simulink model "SystemModel"  (Simulink 8.6)
settings: Solver=ode45  StartTime=0.0  StopTime=25  RelTol=1e-3
values from neighbouring files (symbols this model uses):
  Alt = [ 00  03  03  18  18  05  00  00 ... (first row only)    [constants.m]
  ControlDriverGain = 4.8    [setup.m]
  CurrentDriverBias = Vss/2    [setup.m]
  mBackEMF = 1/Kbmm    [setup.m]
  mElecDynDen = [Lmm Rmm]    [setup.m]
  mElecDynNum = [1]    [setup.m]
  mHeliDynDen = [M B1 0]    [setup.m]
  mHeliDynNum = [0 0 1]    [setup.m]
  mMechDynDen = [Jmm+Jmr Bmm+Bmr]    [setup.m]
  mMechDynNum = [RPMPerw / Kgm2Pergcm2]    [setup.m]
  mPID = [0.0446, 0.0497, 0.0388]    [setup.m]
  mSat = Vss/2    [setup.m]
  mTConst = Ktmm    [setup.m]
  potentiometerBias = Vss/2    [setup.m]
  potentiometerGain = Vss/(2*angleRange)    [setup.m]
  tHeliDynDen = [Jh B2h 0] * Kgm2Pergcm2    [setup.m]
  tHeliDynNum = [0 0 1]    [setup.m]
  torqueFromAltMotorMass = (mainBracketMass + Mmm) * G * mainArmLength    [setup.m]
  torqueFromYawMotorMass = (tailBracketMass + Mtm) * G * yawArmLength    [setup.m]
  tSat = Vss/2    [setup.m]
  tTorque = TPtr*1e-6 * G * Lh*1e-2 * Ntr    [setup.m]
  Yaw = [ 00  00  60  60 180 180 ... (first row only)    [constants.m]
undefined symbols (not defined in the file or in its folder): mLift
libraries: simulink x4, vrlib x1, simulink_extras x1
settings Model: Creator=Leos  LastModifiedBy=Wyatt
settings DataIOCC: LimitDataPoints=off
settings DebuggingCC: FcnCallInpInsideContextMsg=UseLocalSettings
settings ConfigComp: CovSFcnEnable=off

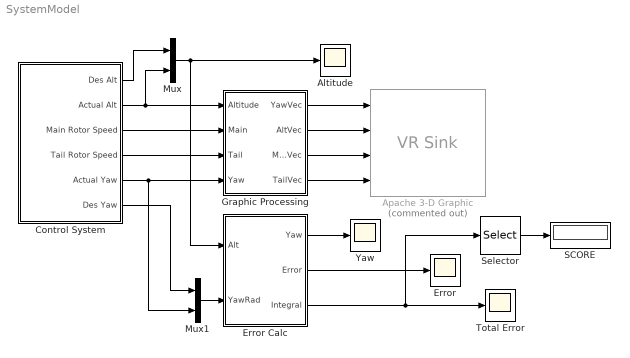
== system SystemModel ==
  Altitude : Scope
  Apache 3-D Graphic : vrlib/VR Sink  Commented=on  InstantiateOnLoad=on  SampleTime=-1  ViewEnable=on  RemoteChange=off  RemoteView=off  FieldsWritten=Helicopter.rotation.4.1.double#Helicopter.translation.3.1.double#Main.rotation.4.1.double#Tail.rotation.4.1.double  WorldFileName=Apache.WRL  AutoView=on  VideoDimensions=[]  AllowVariableSize=off  FigureProperties="{'Position', 'Name', 'Viewpoint', 'CameraBound', 'CameraDirection', 'CameraPosition', 'CameraUpVector', 'ZoomFactor', 'Antialiasing', 'Headlight', 'Lighting', 'NavPanel', 'Sound', 'StatusBar', 'Stereo3D', 'Stereo3DCameraOffset', 'Stereo3DHIT', 'ToolBar', 'Textures', 'Transparency', 'Triad', 'Wireframe', 'NavZones', 'NavMode', 'NavSpeed', 'CaptureFileFormat', 'CaptureFileName', 'Record2DCompressMethod', 'Record2DCompressQuality', 'Record2D', 'Record2DFileName', 'Record2DFPS'; [2.7530000000000000e+03  -5.1800000000000000e+02   5.7600000000000000e+02   3.8000000000000000e+02], '', '_untitled_1', 'on', [0.0000000000000000e+00   0.0000000000000000e+00  -1.0000000000000000e+00], [0.0000000000000000e+00   0.0000000000000000e+00   0.0000000000000000e+00], [0.0000000000000000e+00   1.0000000000000000e+00   0.0000000000000000e+00], [1.0000000000000000e+00], 'on', 'on', 'on', 'halfbar', 'on', 'on', 'off', [1.0000000149011612e-01], [0.0000000000000000e+00], 'on', 'on', 'on', 'none', 'off', 'off', 'walk', 'normal', 'tif', '%f_anim_%n.tif', 'auto', [7.5000000000000000e+01], 'off', '%f_anim_%n.avi', 'auto'}"
  Control System : Subsystem
  Error : Scope
  Error Calc : Subsystem
  Graphic Processing : Subsystem
  Mux : Mux  Inputs=2
  Mux1 : Mux  Inputs=2
  SCORE : Display
  Selector : Selector  InputPortWidth=3  IndexOptions=Index vector (dialog)  Indices=[3]  OutputSizes=1
  Total Error : Scope
  Yaw : Scope
  wires:
  Mux/1 -> Error Calc/1(Alt), Altitude/1
  Control System/1(Des Alt) -> Mux/1
  Control System/2(Actual Alt) -> Mux/2, Graphic Processing/1(Altitude)
  Control System/5(Actual Yaw) -> Mux1/2, Graphic Processing/4(Yaw)
  Graphic Processing/1(YawVec) -> Apache 3-D Graphic/1
  Graphic Processing/2(AltVec) -> Apache 3-D Graphic/2
  Graphic Processing/3(MainVec) -> Apache 3-D Graphic/3
  Graphic Processing/4(TailVec) -> Apache 3-D Graphic/4
  Control System/4(Tail Rotor Speed) -> Graphic Processing/3(Tail)
  Control System/3(Main Rotor Speed) -> Graphic Processing/2(Main)
  Control System/6(Des Yaw) -> Mux1/1
  Mux1/1 -> Error Calc/2(YawRad)
  Error Calc/1(Yaw) -> Yaw/1
  Error Calc/2(Error) -> Error/1
  Error Calc/3(Integral) -> Selector/1, Total Error/1
  Selector/1 -> SCORE/1

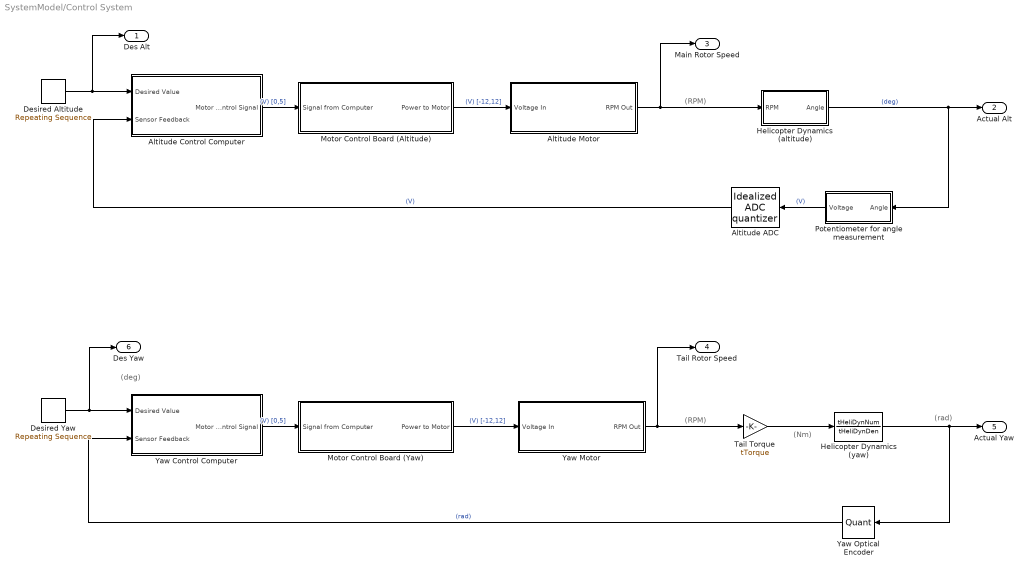
== system SystemModel/Control System ==
  note: (RPM)
  note: (deg)
  note: (RPM)
  note: (Nm)
  note: (rad)
  Altitude ADC : simulink_extras/Additional Discrete/Idealized ADC quantizer  NumberOfConverterBits=ADC_bitwidth  Vmin=ground  Vmax=Vss  OutputDataType=int16  OutputNegativeValues=off
  Altitude Control Computer : Subsystem
  Altitude Motor : Subsystem
  Desired Altitude : simulink/Sources/Repeating Sequence  rep_seq_t=Alt(2,:)  rep_seq_y=Alt(1,:)
  Desired Yaw : simulink/Sources/Repeating Sequence  rep_seq_t=Yaw(2,:)  rep_seq_y=Yaw(1,:)
  Helicopter Dynamics (yaw) : TransferFcn  Numerator=tHeliDynNum  Denominator=tHeliDynDen
  Helicopter Dynamics (altitude) : Subsystem
  Motor Control Board (Altitude) : Subsystem
  Motor Control Board (Yaw) : Subsystem
  Potentiometer for angle measurement : Subsystem
  Tail Torque : Gain  Gain=tTorque
  Yaw Control Computer : Subsystem
  Yaw Motor : Subsystem
  Yaw Optical Encoder : Quantizer  QuantizationInterval=YawEncoderQuantization
  Des Alt : Outport
  Actual Alt : Outport  Port=2
  Main Rotor Speed : Outport  Port=3
  Tail Rotor Speed : Outport  Port=4
  Actual Yaw : Outport  Port=5
  Des Yaw : Outport  Port=6
  wires:
  Desired Altitude/1 -> Altitude Control Computer/1(Desired Value), Des Alt/1
  Tail Torque/1 -> Helicopter Dynamics (yaw)/1
  Helicopter Dynamics (yaw)/1 -> Yaw Optical Encoder/1, Actual Yaw/1
  Desired Yaw/1 -> Yaw Control Computer/1(Desired Value), Des Yaw/1
  Altitude Motor/1(RPM Out) -> Helicopter Dynamics (altitude)/1(RPM), Main Rotor Speed/1
  Yaw Optical Encoder/1 -> Yaw Control Computer/2(Sensor Feedback)  "(rad)"
  Yaw Control Computer/1(Motor Driver Control Signal) -> Motor Control Board (Yaw)/1(Signal from Computer)  "(V) [0,5]"
  Altitude Control Computer/1(Motor Driver Control Signal) -> Motor Control Board (Altitude)/1(Signal from Computer)  "(V) [0,5]"
  Motor Control Board (Altitude)/1(Power to Motor) -> Altitude Motor/1(Voltage In)  "(V) [-12,12]"
  Motor Control Board (Yaw)/1(Power to Motor) -> Yaw Motor/1(Voltage In)  "(V) [-12,12]"
  Yaw Motor/1(RPM Out) -> Tail Torque/1, Tail Rotor Speed/1
  Altitude ADC/1 -> Altitude Control Computer/2(Sensor Feedback)  "(V)"
  Potentiometer for angle measurement/1(Voltage) -> Altitude ADC/1  "(V)"
  Helicopter Dynamics (altitude)/1(Angle) -> Actual Alt/1, Potentiometer for angle measurement/1(Angle)  "(deg)"

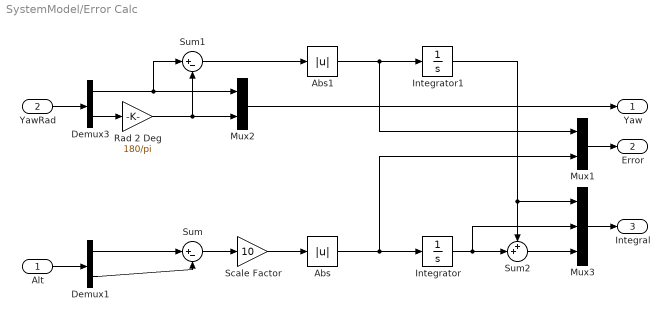
== system SystemModel/Error Calc ==
  Alt : Inport
  YawRad : Inport  Port=2
  Abs : Abs
  Abs1 : Abs
  Demux1 : Demux  Outputs=2
  Demux3 : Demux  Outputs=2
  Integrator : Integrator
  Integrator1 : Integrator
  Mux1 : Mux  Inputs=2
  Mux2 : Mux  Inputs=2
  Mux3 : Mux  Inputs=3
  Rad 2 Deg : Gain  Gain=180/pi
  Scale Factor : Gain  Gain=10
  Sum : Sum  Inputs=|+-
  Sum1 : Sum  Inputs=|+-
  Sum2 : Sum  Inputs=++|
  Yaw : Outport
  Error : Outport  Port=2
  Integral : Outport  Port=3
  wires:
  YawRad/1 -> Demux3/1
  Alt/1 -> Demux1/1
  Mux2/1 -> Yaw/1
  Rad 2 Deg/1 -> Sum1/2, Mux2/2
  Demux3/2 -> Rad 2 Deg/1
  Demux3/1 -> Sum1/1, Mux2/1
  Demux1/1 -> Sum/1
  Demux1/2 -> Sum/2
  Sum/1 -> Scale Factor/1
  Mux1/1 -> Error/1
  Sum1/1 -> Abs1/1
  Abs1/1 -> Mux1/1, Integrator1/1
  Scale Factor/1 -> Abs/1
  Abs/1 -> Mux1/2, Integrator/1
  Mux3/1 -> Integral/1
  Integrator/1 -> Mux3/2, Sum2/2
  Integrator1/1 -> Mux3/1, Sum2/1
  Sum2/1 -> Mux3/3

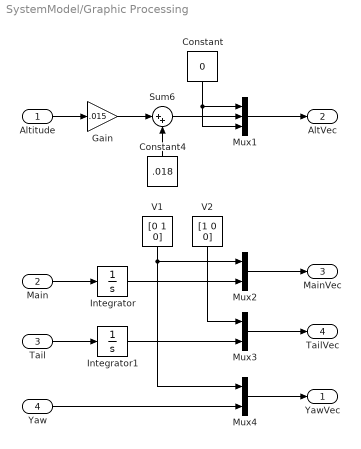
== system SystemModel/Graphic Processing ==
  Altitude : Inport
  Main : Inport  Port=2
  Tail : Inport  Port=3
  Yaw : Inport  Port=4
  Constant : Constant  Value=0
  Constant4 : Constant  Value=.018
  Gain : Gain  Gain=.015
  Integrator : Integrator
  Integrator1 : Integrator
  Mux1 : Mux  Inputs=3
  Mux2 : Mux  Inputs=2
  Mux3 : Mux  Inputs=2
  Mux4 : Mux  Inputs=2
  Sum6 : Sum  Inputs=|++
  V1 : Constant  Value=[0 1 0]
  V2 : Constant  Value=[1 0 0]
  YawVec : Outport
  AltVec : Outport  Port=2
  MainVec : Outport  Port=3
  TailVec : Outport  Port=4
  wires:
  V2/1 -> Mux3/1
  Yaw/1 -> Mux4/2
  Altitude/1 -> Gain/1
  Constant4/1 -> Sum6/2
  Sum6/1 -> Mux1/2
  Gain/1 -> Sum6/1
  Mux4/1 -> YawVec/1
  Mux3/1 -> TailVec/1
  Tail/1 -> Integrator1/1
  Mux2/1 -> MainVec/1
  Mux1/1 -> AltVec/1
  V1/1 -> Mux4/1, Mux2/1
  Main/1 -> Integrator/1
  Constant/1 -> Mux1/3, Mux1/1
  Integrator/1 -> Mux2/2
  Integrator1/1 -> Mux3/2

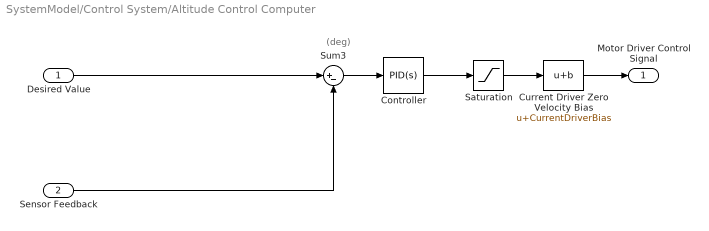
== system SystemModel/Control System/Altitude Control Computer ==
  note: (deg)
  Desired Value : Inport
  Sensor Feedback : Inport  Port=2
  Controller : simulink/Continuous/PID Controller  Controller=PID  TimeDomain=Continuous-time  SampleTime=-1  IntegratorMethod=Forward Euler  FilterMethod=Forward Euler  Form=Parallel  UseFilter=on  ControllerParametersSource=internal  P=mPID(1)  I=mPID(2)  D=mPID(3)  N=100  InitialConditionSource=internal  InitialConditionForIntegrator=0  InitialConditionForFilter=0  ExternalReset=none  LimitOutput=off  UpperSaturationLimit=inf  LowerSaturationLimit=-inf  LinearizeAsGain=on  AntiWindupMode=none  Kb=1  TrackingMode=off  Kt=1  PParamMin=[]  PParamMax=[]  IParamMin=[]  IParamMax=[]  DParamMin=[]  DParamMax=[]  NParamMin=[]  NParamMax=[]  KbParamMin=[]  KbParamMax=[]  KtParamMin=[]  KtParamMax=[]  POutMin=[]  POutMax=[]  IOutMin=[]  IOutMax=[]  DOutMin=[]  DOutMax=[]  NOutMin=[]  NOutMax=[]  KbOutMin=[]  KbOutMax=[]  KtOutMin=[]  KtOutMax=[]  IntegratorOutMin=[]  IntegratorOutMax=[]  FilterOutMin=[]  FilterOutMax=[]  SumOutMin=[]  SumOutMax=[]  SumI1OutMin=[]  SumI1OutMax=[]  SumI2OutMin=[]  SumI2OutMax=[]  SumI3OutMin=[]  SumI3OutMax=[]  SumDOutMin=[]  SumDOutMax=[]  SaturationOutMin=[]  SaturationOutMax=[]  IntegratorContinuousStateAttributes=''  IntegratorStateMustResolveToSignalObject=off  IntegratorRTWStateStorageClass=Auto  FilterContinuousStateAttributes=''  FilterStateMustResolveToSignalObject=off  FilterRTWStateStorageClass=Auto  DifferentiatorICPrevScaledInput=0  DifferentiatorOutMin=[]  DifferentiatorOutMax=[]
  Current Driver Zero Velocity Bias : Bias  Bias=CurrentDriverBias
  Saturation : Saturate  UpperLimit=mSat  LowerLimit=-mSat
  Sum3 : Sum  Inputs=|+-
  Motor Driver Control Signal : Outport
  wires:
  Desired Value/1 -> Sum3/1
  Sensor Feedback/1 -> Sum3/2
  Sum3/1 -> Controller/1
  Saturation/1 -> Current Driver Zero Velocity Bias/1
  Controller/1 -> Saturation/1
  Current Driver Zero Velocity Bias/1 -> Motor Driver Control Signal/1

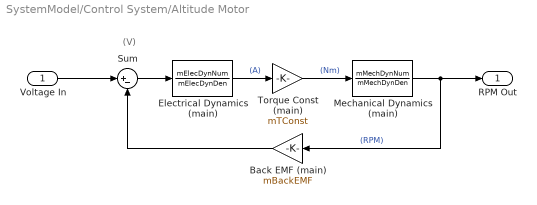
== system SystemModel/Control System/Altitude Motor ==
  note: (V)
  Voltage In : Inport
  Back EMF (main) : Gain  Gain=mBackEMF
  Electrical Dynamics (main) : TransferFcn  Numerator=mElecDynNum  Denominator=mElecDynDen
  Mechanical Dynamics (main) : TransferFcn  Numerator=mMechDynNum  Denominator=mMechDynDen
  Sum : Sum  Inputs=|+-
  Torque Const (main) : Gain  Gain=mTConst
  RPM Out : Outport
  wires:
  Voltage In/1 -> Sum/1
  Torque Const (main)/1 -> Mechanical Dynamics (main)/1  "(Nm)"
  Back EMF (main)/1 -> Sum/2
  Mechanical Dynamics (main)/1 -> RPM Out/1, Back EMF (main)/1  "(RPM)"
  Electrical Dynamics (main)/1 -> Torque Const (main)/1  "(A)"
  Sum/1 -> Electrical Dynamics (main)/1

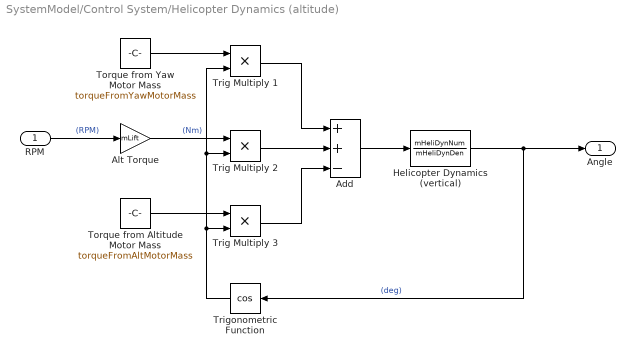
== system SystemModel/Control System/Helicopter Dynamics (altitude) ==
  RPM : Inport
  Add : Sum  Inputs=++-
  Alt Torque : Gain  Gain=mLift
  Helicopter Dynamics (vertical) : TransferFcn  Numerator=mHeliDynNum  Denominator=mHeliDynDen
  Torque from Altitude Motor Mass : Constant  Value=torqueFromAltMotorMass
  "Torque from Yaw Motor Mass " : Constant  Value=torqueFromYawMotorMass
  Trig Multiply 1 : Product
  Trig Multiply 2 : Product
  Trig Multiply 3 : Product
  Trigonometric Function : Trigonometry  Operator=cos
  Angle : Outport
  wires:
  RPM/1 -> Alt Torque/1  "(RPM)"
  Helicopter Dynamics (vertical)/1 -> Angle/1, Trigonometric Function/1  "(deg)"
  Alt Torque/1 -> Trig Multiply 2/1  "(Nm)"
  Trigonometric Function/1 -> Trig Multiply 3/2, Trig Multiply 2/2, Trig Multiply 1/2
  "Torque from Yaw Motor Mass "/1 -> Trig Multiply 1/1
  Add/1 -> Helicopter Dynamics (vertical)/1
  Trig Multiply 2/1 -> Add/2
  Trig Multiply 1/1 -> Add/1
  Torque from Altitude Motor Mass/1 -> Trig Multiply 3/1
  Trig Multiply 3/1 -> Add/3

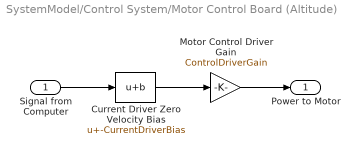
== system SystemModel/Control System/Motor Control Board (Altitude) ==
  Signal from Computer : Inport
  Current Driver Zero Velocity Bias : Bias  Bias=-CurrentDriverBias
  Motor Control Driver Gain : Gain  Gain=ControlDriverGain
  Power to Motor : Outport
  wires:
  Motor Control Driver Gain/1 -> Power to Motor/1
  Signal from Computer/1 -> Current Driver Zero Velocity Bias/1
  Current Driver Zero Velocity Bias/1 -> Motor Control Driver Gain/1

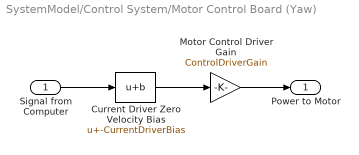
== system SystemModel/Control System/Motor Control Board (Yaw) ==
  Signal from Computer : Inport
  Current Driver Zero Velocity Bias : Bias  Bias=-CurrentDriverBias
  Motor Control Driver Gain : Gain  Gain=ControlDriverGain
  Power to Motor : Outport
  wires:
  Motor Control Driver Gain/1 -> Power to Motor/1
  Signal from Computer/1 -> Current Driver Zero Velocity Bias/1
  Current Driver Zero Velocity Bias/1 -> Motor Control Driver Gain/1

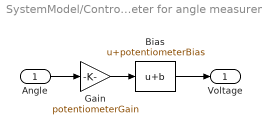
== system SystemModel/Control System/Potentiometer for angle measurement ==
  Angle : Inport
  Bias : Bias  Bias=potentiometerBias
  Gain : Gain  Gain=potentiometerGain
  Voltage : Outport
  wires:
  Bias/1 -> Voltage/1
  Angle/1 -> Gain/1
  Gain/1 -> Bias/1

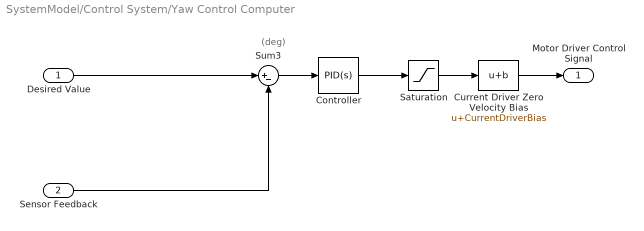
== system SystemModel/Control System/Yaw Control Computer ==
  note: (deg)
  Desired Value : Inport
  Sensor Feedback : Inport  Port=2
  Controller : simulink/Continuous/PID Controller  Controller=PID  TimeDomain=Continuous-time  SampleTime=-1  IntegratorMethod=Forward Euler  FilterMethod=Forward Euler  Form=Parallel  UseFilter=on  ControllerParametersSource=internal  P=mPID(1)  I=mPID(2)  D=mPID(3)  N=100  InitialConditionSource=internal  InitialConditionForIntegrator=0  InitialConditionForFilter=0  ExternalReset=none  LimitOutput=off  UpperSaturationLimit=inf  LowerSaturationLimit=-inf  LinearizeAsGain=on  AntiWindupMode=none  Kb=1  TrackingMode=off  Kt=1  PParamMin=[]  PParamMax=[]  IParamMin=[]  IParamMax=[]  DParamMin=[]  DParamMax=[]  NParamMin=[]  NParamMax=[]  KbParamMin=[]  KbParamMax=[]  KtParamMin=[]  KtParamMax=[]  POutMin=[]  POutMax=[]  IOutMin=[]  IOutMax=[]  DOutMin=[]  DOutMax=[]  NOutMin=[]  NOutMax=[]  KbOutMin=[]  KbOutMax=[]  KtOutMin=[]  KtOutMax=[]  IntegratorOutMin=[]  IntegratorOutMax=[]  FilterOutMin=[]  FilterOutMax=[]  SumOutMin=[]  SumOutMax=[]  SumI1OutMin=[]  SumI1OutMax=[]  SumI2OutMin=[]  SumI2OutMax=[]  SumI3OutMin=[]  SumI3OutMax=[]  SumDOutMin=[]  SumDOutMax=[]  SaturationOutMin=[]  SaturationOutMax=[]  IntegratorContinuousStateAttributes=''  IntegratorStateMustResolveToSignalObject=off  IntegratorRTWStateStorageClass=Auto  FilterContinuousStateAttributes=''  FilterStateMustResolveToSignalObject=off  FilterRTWStateStorageClass=Auto  DifferentiatorICPrevScaledInput=0  DifferentiatorOutMin=[]  DifferentiatorOutMax=[]
  Current Driver Zero Velocity Bias : Bias  Bias=CurrentDriverBias
  Saturation : Saturate  UpperLimit=tSat  LowerLimit=-tSat
  Sum3 : Sum  Inputs=|+-
  Motor Driver Control Signal : Outport
  wires:
  Desired Value/1 -> Sum3/1
  Sensor Feedback/1 -> Sum3/2
  Sum3/1 -> Controller/1
  Saturation/1 -> Current Driver Zero Velocity Bias/1
  Controller/1 -> Saturation/1
  Current Driver Zero Velocity Bias/1 -> Motor Driver Control Signal/1

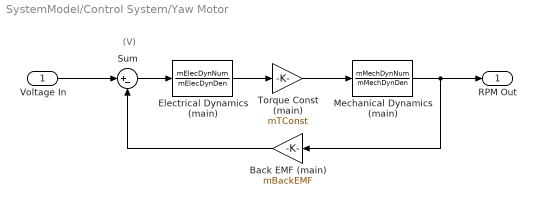
== system SystemModel/Control System/Yaw Motor ==
  note: (V)
  Voltage In : Inport
  Back EMF (main) : Gain  Gain=mBackEMF
  Electrical Dynamics (main) : TransferFcn  Numerator=mElecDynNum  Denominator=mElecDynDen
  Mechanical Dynamics (main) : TransferFcn  Numerator=mMechDynNum  Denominator=mMechDynDen
  Sum : Sum  Inputs=|+-
  Torque Const (main) : Gain  Gain=mTConst
  RPM Out : Outport
  wires:
  Voltage In/1 -> Sum/1
  Torque Const (main)/1 -> Mechanical Dynamics (main)/1
  Back EMF (main)/1 -> Sum/2
  Mechanical Dynamics (main)/1 -> RPM Out/1, Back EMF (main)/1
  Electrical Dynamics (main)/1 -> Torque Const (main)/1
  Sum/1 -> Electrical Dynamics (main)/1
